simulink model "ex3"  (R2021b)
settings: Solver=VariableStepAuto  StartTime=0.0  StopTime=120  RelTol=1e-3
libraries: eeStairGenerator x1
settings Model: Creator=evely  LastModifiedBy=evely

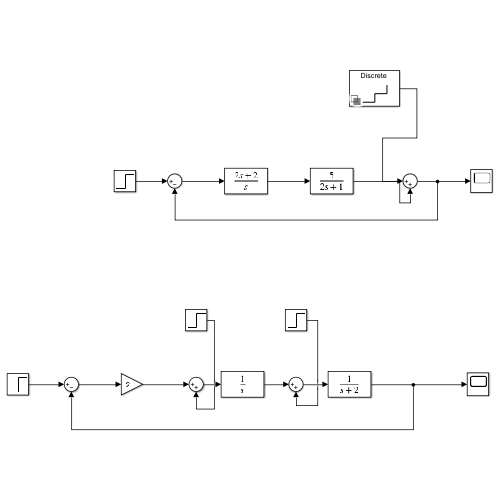
[thumbnail: Simulink's stored preview of the top-level diagram]
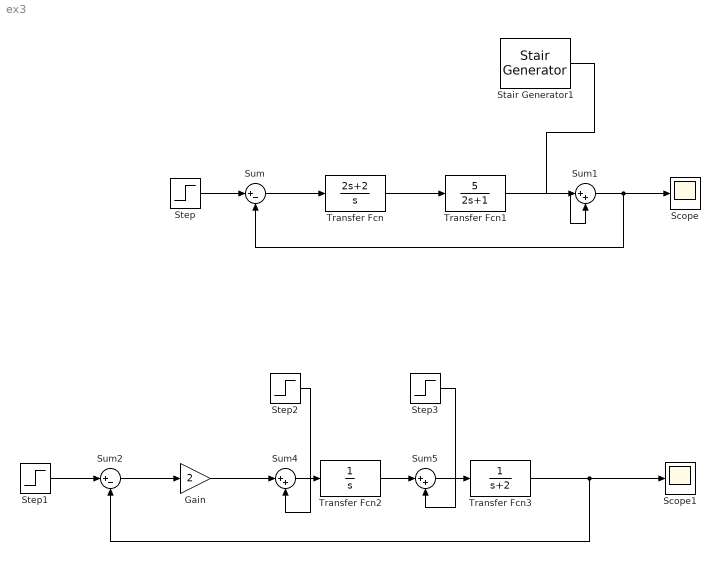
== system ex3 ==
  Gain : Gain  Gain=2
  Scope : Scope
  Scope1 : Scope
  Stair Generator1 : eeStairGenerator/Stair Generator  LabelModeActiveChoice=Discrete  TimeInput=[10 20 30]  AmplitudeInput=[0.2 0.3 0.4]  SampleTime=0.1  RepeatPattern=off  OutDataTypeStr=double
      settings: SourceProductBaseCode=PS
  Step : Step  Time=0  SampleTime=0
  Step1 : Step  Time=0  SampleTime=0
  Step2 : Step  Time=40  SampleTime=0
  Step3 : Step  Time=80  SampleTime=0
  Sum : Sum  Inputs=|+-
  Sum1 : Sum  Inputs=|++
  Sum2 : Sum  Inputs=|+-
  Sum4 : Sum  Inputs=|++
  Sum5 : Sum  Inputs=|++
  Transfer Fcn : TransferFcn  Numerator=[2 2]  Denominator=[1 0]
  Transfer Fcn1 : TransferFcn  Numerator=[5]  Denominator=[2 1]
  Transfer Fcn2 : TransferFcn  Denominator=[1 0]
  Transfer Fcn3 : TransferFcn  Denominator=[1 2]
  wires:
  Transfer Fcn/1 -> Transfer Fcn1/1
  Sum/1 -> Transfer Fcn/1
  Step/1 -> Sum/1
  Transfer Fcn1/1 -> Sum1/2
  Stair Generator1/1 -> Sum1/1
  Sum1/1 -> Sum/2, Scope/1
  Step1/1 -> Sum2/1
  Gain/1 -> Sum4/1
  Sum4/1 -> Transfer Fcn2/1
  Transfer Fcn2/1 -> Sum5/1
  Sum5/1 -> Transfer Fcn3/1
  Step3/1 -> Sum5/2
  Transfer Fcn3/1 -> Sum2/2, Scope1/1
  Step2/1 -> Sum4/2
  Sum2/1 -> Gain/1
